simulink model "pendulo"  (Simulink 8.5)
settings: Solver=ode45  StartTime=0.0  StopTime=10.0  RelTol=1e-3
values from neighbouring files (symbols this model uses):
  l = num2str(l)    [pend.m]
  m = num2str(m)    [pend.m]
undefined symbols (not defined in the file or in its folder): g, sen
settings Model: Creator=Dinis  LastModifiedBy=Dinis  CovModelRefEnable=off
settings DataIOCC: LimitDataPoints=off  SaveFormat=Dataset  SignalLoggingSaveFormat=Dataset
settings OptimizationCC: ExpressionDepthLimit=128
settings DebuggingCC: UnderspecifiedInitializationDetection=Simplified  MergeDetectMultiDrivingBlocksExec=error  FcnCallInpInsideContextMsg=EnableAllAsError  StateNameClashWarn=none
settings HardwareCC: ProdBitPerPointer=64  ProdLargestAtomicFloat=Float  ProdIntDivRoundTo=Zero  ProdEndianess=LittleEndian  ProdHWDeviceType=Specified
settings ModelReferenceCC: PropagateSignalLabelsOutOfModel=on
settings GRTTargetCC: CombineOutputUpdateFcns=on  GRTInterface=off

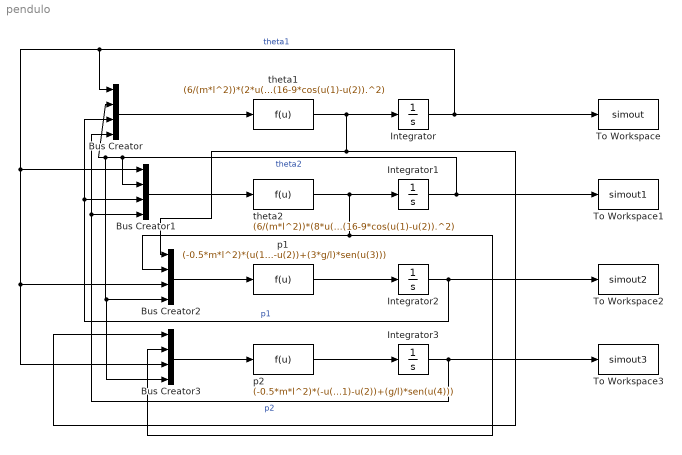
== system pendulo ==
  Bus Creator{,1..3} (4 alike) : BusCreator  Inputs=4
  Integrator{,1..3} (4 alike) : Integrator
  To Workspace : ToWorkspace  VariableName=simout  SaveFormat=Timeseries  SampleTime=-1
  To Workspace1 : ToWorkspace  VariableName=simout1  SaveFormat=Timeseries  SampleTime=-1
  To Workspace2 : ToWorkspace  VariableName=simout2  SaveFormat=Timeseries  SampleTime=-1
  To Workspace3 : ToWorkspace  VariableName=simout3  SaveFormat=Timeseries  SampleTime=-1
  p1 : Fcn  Expr=(-0.5*m*l^2)*(u(1)*u(2)*sen(u(1)-u(2))+(3*g/l)*sen(u(3)))
  p2 : Fcn  Expr=(-0.5*m*l^2)*(-u(1)*u(2)*sen(u(1)-u(2))+(g/l)*sen(u(4)))
  theta1 : Fcn  Expr=(6/(m*l^2))*(2*u(3)-3*cos(u(1)-u(2))*u(4))/(16-9*cos(u(1)-u(2)).^2)
  theta2 : Fcn  Expr=(6/(m*l^2))*(8*u(4)-3*cos(u(1)-u(2))*u(3))/(16-9*cos(u(1)-u(2)).^2)
  wires:
  p1/1 -> Integrator2/1
  p2/1 -> Integrator3/1
  Bus Creator/1 -> theta1/1
  Integrator1/1 -> To Workspace1/1, Bus Creator1/2, Bus Creator3/4, Bus Creator2/4, Bus Creator/2  "theta2"
  Integrator2/1 -> To Workspace2/1, Bus Creator1/3, Bus Creator/3  "p1"
  Integrator3/1 -> To Workspace3/1, Bus Creator1/4, Bus Creator/4  "p2"
  Integrator/1 -> To Workspace/1, Bus Creator/1, Bus Creator3/3, Bus Creator2/3, Bus Creator1/1  "theta1"
  Bus Creator1/1 -> theta2/1
  Bus Creator3/1 -> p2/1
  Bus Creator2/1 -> p1/1
  theta1/1 -> Bus Creator3/1, Bus Creator2/1, Integrator/1
  theta2/1 -> Bus Creator3/2, Bus Creator2/2, Integrator1/1
